simulink model "s_3dgyro_lqr"  (Simulink 8.0)
settings: Solver=ode1  StartTime=0.0  StopTime=inf  FixedStep=0.004  RelTol=1e-3
values from neighbouring files (symbols this model uses):
  A = [0 0 -h/Jy 0; 0 0 1 0; h/Jz 0 0 0; 0 1 0 0]    [setup_3dgyro.m]
  B = [1/Jy; 0; 0; 0]    [setup_3dgyro.m]
  K = lqr(A,B,Q,R)    [setup_3dgyro.m]
settings Model: Creator=ajavid  LastModifiedBy=pmartin  SimulationMode=external  ExtModeTrigDuration=100000
settings SolverCC: PositivePriorityOrder=on
settings DataIOCC: SignalLoggingSaveFormat=ModelDataLogs
settings OptimizationCC: InitFltsAndDblsToZero=on
settings DebuggingCC: MultiTaskDSMMsg=warning  MultiTaskCondExecSysMsg=none  FcnCallInpInsideContextMsg=UseLocalSettings  StrictBusMsg=None
settings HardwareCC: TargetHWDeviceType=32-bit Generic
settings RTWCC: SystemTargetFile=quarc_windows.tlc  TemplateMakefile=quarc_default_tmf  Description=QuaRC Win32 Target  ProcessScript=quarc_windows_make_rtw_hook  IncludeERTFirstTime=on
settings STFCustomTargetCC: TargetFcnLib=ansi_tfl_tmw.mat  TargetPreCompLibLocation=C:\PROGRA~2\QUARC\lib\2012b\windows\release  CodeReplacementLibrary=ANSI_C  GeneratePreprocessorConditionals=Disable all  SystemTargetFile=quarc_windows.tlc
settings GRTTargetCC: TargetFcnLib=ansi_tfl_tmw.mat  TargetPreCompLibLocation=C:\PROGRA~2\QUARC\lib\2012b\windows\release  ParMdlRefBuildCompliant=off  CompOptLevelCompliant=off  ConcurrentExecutionCompliant=off  CombineOutputUpdateFcns=off  MatFileLogging=off  GRTInterface=on  ExtMode=on  ExtModeMexFile=quarc_comm

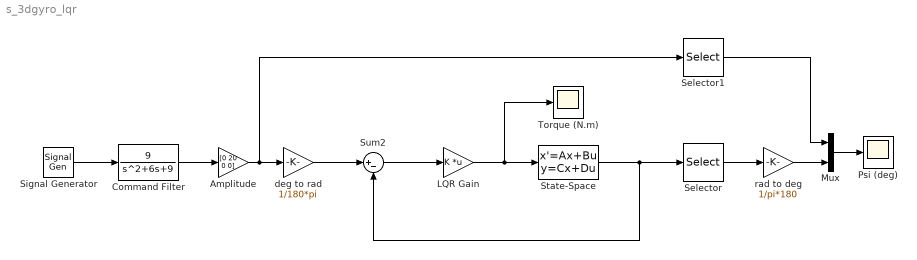
== system s_3dgyro_lqr ==
  Amplitude : Gain  Gain=[0 20 0 0]
  Command Filter : TransferFcn  Numerator=[9]  Denominator=[1 6 9]
  LQR Gain : Gain  Gain=K  Multiplication=Matrix(K*u)
  Mux : Mux  Inputs=2
  Psi (deg) : Scope
      settings: YMin=-30  YMax=30  SaveName=Psi  MaxDataPoints=250000
  Selector : Selector  InputPortWidth=4  IndexOptions=Index vector (dialog)  Indices=2  OutputSizes=1
  Selector1 : Selector  InputPortWidth=4  IndexOptions=Index vector (dialog)  Indices=2  OutputSizes=1
  Signal Generator : SignalGenerator  WaveForm=square  Frequency=0.1
  State-Space : StateSpace  A=A  B=B  C=eye(4)  D=zeros(4,1)  X0=[0 0 0 0]
  Sum2 : Sum  Inputs=|+-
  Torque (N.m) : Scope
      settings: YMin=-0.3  YMax=0.3
  deg to rad : Gain  Gain=1/180*pi
  rad to deg : Gain  Gain=1/pi*180
  wires:
  Command Filter/1 -> Amplitude/1
  deg to rad/1 -> Sum2/1
  Sum2/1 -> LQR Gain/1
  LQR Gain/1 -> Torque (N.m)/1, State-Space/1
  Signal Generator/1 -> Command Filter/1
  Amplitude/1 -> Selector1/1, deg to rad/1
  State-Space/1 -> Sum2/2, Selector/1
  Selector/1 -> rad to deg/1
  rad to deg/1 -> Mux/2
  Mux/1 -> Psi (deg)/1
  Selector1/1 -> Mux/1
